simulink model "History1"  (Simulink 5.0)
settings: Solver=ode45  StartTime=0.0  StopTime=10.0  RelTol=1e-3
settings Model: Creator=scaife  LastModifiedBy=scaife  ExtModeAutoUpdateStatusClock=off

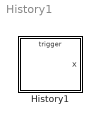
== system History1 ==
  History1 : Stateflow chart

== stateflow chart History1 ==
  state A
    (history)
    state A1/
      en: x+=1;
      ex: x-=1;
    state A2/
      en: x+=10;
      ex: x-=10;
    A1 -> A2 : E
    A2 -> A1 : E
    (default) -> A1
  state B
    (history)
    state B1/
      en: x+=100;
      ex: x-=100;
    state B2/
      en: x+=1000;
      ex: x-=1000;
    (default) -> B1
    B2 -> B1 : E
    B1 -> B2 : E
  (default) -> A
  A -> B : F
  B -> A : F
  data: x output int32
  events: E input EITHER_EDGE_EVENT; F input EITHER_EDGE_EVENT
